simulink model "Simple_4Quad_payload_08_2017b"  (R2017b)
settings: Solver=ode45  StartTime=0.0  StopTime=200  RelTol=1e-3
InitFcn:
  | Simple_4Quad_payload_08_const
values from neighbouring files (symbols this model uses):
  All_rho = [d1 0 0 ... (first row only)    [Colab_4Quad_model_01_const.m]    (also in Colab_4Quad_model_02_const.m; Simple_4Quad_payload_04_const.m; Simple_4Quad_payload_05_const.m; Simple_4Quad_payload_06_const.m)
  alphaTF = 0.1    [Simple_4Quad_payload_08_const.m]    (also in Simple_4Quad_payload_09_const.m = 0.5; Simple_4Quad_payload_10_const.m = 1; Simple_4Quad_payload_11_const.m = 0.5; Simple_4Quad_payload_12_const.m = 10)
  B_ob = [zeros(3);eye(3)]    [Simple_4Quad_payload_04_const.m]    (also in Simple_4Quad_payload_05_const.m; Simple_4Quad_payload_06_const.m; Simple_4Quad_payload_07_const.m; Simple_4Quad_payload_08_const.m)
  BBT_inv = ((B'*B)^(-1))*B'    [Simple_2Quad_payload_03_const.m]    (also in Simple_4Quad_payload_04_const.m = ((BR'*BR)^(-1))*BR'; Simple_4Quad_payload_05_const.m = ((BR'*BR)^(-1))*BR'; Simple_4Quad_payload_06_const.m = ((BR'*BR)^(-1))*BR'; Simple_4Quad_payload_07_const.m = ((BR'*BR)^(-1))*BR')
  BR = 1e0*eye(n)    [Simple_4Quad_payload_04_const.m]    (also in Simple_4Quad_payload_05_const.m; Simple_4Quad_payload_06_const.m; Simple_4Quad_payload_07_const.m; Simple_4Quad_payload_08_const.m)
  C_ob = [eye(3) zeros(3)]    [Simple_4Quad_payload_04_const.m]    (also in Simple_4Quad_payload_05_const.m; Simple_4Quad_payload_06_const.m; Simple_4Quad_payload_07_const.m; Simple_4Quad_payload_08_const.m)
  d1 = 0.25    [Colab_4Quad_model_01_const.m]    (also in Colab_4Quad_model_02_const.m = 0.5; Simple_4Quad_payload_01_const.m = 1; Simple_4Quad_payload_02_const.m = 1; Simple_4Quad_payload_03_const.m = 1)
  d2 = 0.25    [Colab_4Quad_model_01_const.m]    (also in Colab_4Quad_model_02_const.m = 0.5; Simple_4Quad_payload_01_const.m = 1; Simple_4Quad_payload_02_const.m = 1; Simple_4Quad_payload_03_const.m = 1)
  Des_rel_dist = 2    [Simple_4Quad_payload_01_const.m]    (also in Simple_4Quad_payload_02_const.m = 4; Simple_4Quad_payload_03_const.m = 4; Simple_4Quad_payload_04_const.m; Simple_4Quad_payload_05_const.m)
  g = 9.81    [Colab_4Quad_model_01_const.m]    (also in Colab_4Quad_model_02_const.m; Simple_2Quad_payload_01_const.m; Simple_2Quad_payload_02_const.m; Simple_2Quad_payload_03_const.m)
  gamma_0 = 1e-0*diag([1e-3;1e-0])    [Simple_2Quad_payload_03_const.m]    (also in Simple_4Quad_payload_04_const.m = 1e-0*diag([1e-6*ones(3,1);1e-0*ones(3,1)]); Simple_4Quad_payload_05_const.m = 1e-1*diag([1e-6*ones(3,1);1e-0*ones(3,1)]); Simple_4Quad_payload_06_const.m = 1e-0*diag([1e-6*ones(3,1);1e-0*ones(3,1)]); Simple_4Quad_payload_07_const.m = 1e-0*diag([1e-6*ones(3,1);1e-0*ones(3,1)]))
  gamma_0L = 1e-0*diag([1e-6*ones(3,1);1e-0*ones(3,1)])    [Simple_4Quad_payload_08_const.m]    (also in Simple_4Quad_payload_09_const.m; Simple_4Quad_payload_10_const.m = 1e+0*diag([1e-3*ones(3,1);1e-3*ones(3,1)]); Simple_4Quad_payload_11_const.m = 1e+0*diag([1e-3*ones(3,1);1e-3*ones(3,1)]); Simple_4Quad_payload_12_const.m = 1e+2*diag(1e-4*ones(3,1)))
  gamma_0o = 1e-6*diag([1e-0*ones(3,1);1e-0*ones(3,1)])    [Simple_4Quad_payload_08_const.m]    (also in Simple_4Quad_payload_09_const.m = 1e-0*diag([1e-3*ones(3,1);1e-3*ones(3,1)]))
  gamma_0v = 1e-0*diag([1e-0*ones(3,1);1e-0*ones(3,1)])    [Simple_4Quad_payload_08_const.m]    (also in Simple_4Quad_payload_09_const.m = 1e-0*diag([1e-6*ones(3,1);1e-6*ones(3,1)]); Simple_4Quad_payload_10_const.m = 1e+0*diag(1e-0*ones(3,1)); Simple_4Quad_payload_11_const.m = 1e+0*diag(1e-0*ones(3,1)); Simple_4Quad_payload_12_const.m = 1e+3*diag(1e-0*ones(3,1)))
  gamma_1 = 1e+2*diag([1e-3;1e-0])    [Simple_2Quad_payload_03_const.m]    (also in Simple_4Quad_payload_04_const.m = 1e+2*diag([1e-6*ones(3,1);1e-0*ones(3,1)]); Simple_4Quad_payload_05_const.m = 1e+2*diag([1e-6*ones(3,1);1e-0*ones(3,1)]); Simple_4Quad_payload_06_const.m = 1e+3*diag([1e-6*ones(3,1);1e-0*ones(3,1)]); Simple_4Quad_payload_07_const.m = 1e+3*diag([1e-6*ones(3,1);1e-0*ones(3,1)]))
  gamma_1L = 1e+3*diag([1e-6*ones(3,1);1e-0*ones(3,1)])    [Simple_4Quad_payload_08_const.m]    (also in Simple_4Quad_payload_09_const.m = 1e+2*diag([1e-6*ones(3,1);1e-0*ones(3,1)]); Simple_4Quad_payload_10_const.m = 1e+1*diag([1e-3*ones(3,1);1e-3*ones(3,1)]); Simple_4Quad_payload_11_const.m = 1e+0*diag([1e-3*ones(3,1);1e-3*ones(3,1)]); Simple_4Quad_payload_12_const.m = 1e+2*diag(1e-4*ones(3,1)))
  gamma_1o = 1e-6*diag([1e-0*ones(3,1);1e-0*ones(3,1)])    [Simple_4Quad_payload_08_const.m]    (also in Simple_4Quad_payload_09_const.m = 1e+2*diag([1e-3*ones(3,1);1e-3*ones(3,1)]))
  gamma_1v = 1e+3*diag([1e-0*ones(3,1);1e-0*ones(3,1)])    [Simple_4Quad_payload_08_const.m]    (also in Simple_4Quad_payload_09_const.m = 1e+2*diag([1e-6*ones(3,1);1e-6*ones(3,1)]); Simple_4Quad_payload_10_const.m = 1e+0*diag(1e-0*ones(3,1)); Simple_4Quad_payload_11_const.m = 1e+0*diag(1e-0*ones(3,1)); Simple_4Quad_payload_12_const.m = 1e+3*diag(1e-0*ones(3,1)))
  Ix = 0.166667    [Colab_4Quad_model_01_const.m]    (also in Colab_4Quad_model_02_const.m = 0.02; Simple_4Quad_payload_01_const.m = 1; Simple_4Quad_payload_02_const.m = 1; Simple_4Quad_payload_03_const.m = 1)
  Iy = 0.166667    [Colab_4Quad_model_01_const.m]    (also in Colab_4Quad_model_02_const.m = 0.02; Simple_4Quad_payload_01_const.m = 1; Simple_4Quad_payload_02_const.m = 1; Simple_4Quad_payload_03_const.m = 1)
  Iz = 0.166667    [Colab_4Quad_model_01_const.m]    (also in Colab_4Quad_model_02_const.m = 0.02; Simple_4Quad_payload_01_const.m = 1; Simple_4Quad_payload_02_const.m = 1; Simple_4Quad_payload_03_const.m = 1)
  Jo = diag([Ix;Iy;Iz])    [Colab_4Quad_model_01_const.m]    (also in Colab_4Quad_model_02_const.m; Simple_4Quad_payload_04_const.m; Simple_4Quad_payload_05_const.m; Simple_4Quad_payload_06_const.m)
  Jq = diag([0.0291 0.0291 0.0552])    [Colab_4Quad_model_01_const.m]    (also in Colab_4Quad_model_02_const.m = diag([0.03 0.03 0.06]); Simple_4Quad_payload_03_const.m = 1.2416e-3 * diag([1 1 2]); Simple_4Quad_payload_04_const.m = 1 * diag([1 1 2]); Simple_4Quad_payload_05_const.m = 1 * diag([1 1 2]))
  k1 = 1    [Simple_2Quad_payload_03_const.m]    (also in Simple_4Quad_payload_04_const.m; Simple_4Quad_payload_05_const.m; Simple_4Quad_payload_06_const.m; Simple_4Quad_payload_07_const.m)
  k2 = 0.1    [Simple_2Quad_payload_03_const.m]    (also in Simple_4Quad_payload_04_const.m; Simple_4Quad_payload_05_const.m; Simple_4Quad_payload_06_const.m; Simple_4Quad_payload_07_const.m)
  l = 3.1819    [Colab_4Quad_model_01_const.m]    (also in Colab_4Quad_model_02_const.m = 3; Simple_2Quad_payload_04_const.m = 1; Simple_4Quad_payload_01_const.m = 1; Simple_4Quad_payload_02_const.m = 2)
  m = 1.5    [Colab_4Quad_model_01_const.m]    (also in Colab_4Quad_model_02_const.m; Simple_2Quad_payload_04_const.m = 1; Simple_4Quad_payload_01_const.m = 1; Simple_4Quad_payload_02_const.m = 1)
  M = 1.0    (= 1)    [Colab_4Quad_model_01_const.m]    (also in Colab_4Quad_model_02_const.m; Simple_2Quad_payload_01_const.m; Simple_2Quad_payload_02_const.m; Simple_2Quad_payload_03_const.m)
  n = 2    [Simple_2Quad_payload_03_const.m]    (also in Simple_4Quad_payload_03_const.m = 6; Simple_4Quad_payload_04_const.m = 6; Simple_4Quad_payload_05_const.m = 6; Simple_4Quad_payload_06_const.m = 6)
  noise_var_Omegao = 0e-6    (= 0)    [Simple_4Quad_payload_07_const.m]    (also in Simple_4Quad_payload_08_const.m; Simple_4Quad_payload_09_const.m; Simple_4Quad_payload_10_const.m; Simple_4Quad_payload_11_const.m)
  noise_var_RelAcc = 0e-6    (= 0)    [Simple_4Quad_payload_07_const.m]    (also in Simple_4Quad_payload_08_const.m; Simple_4Quad_payload_09_const.m; Simple_4Quad_payload_10_const.m; Simple_4Quad_payload_11_const.m)
  noise_var_RelPos = 0e-6    (= 0)    [Simple_4Quad_payload_07_const.m]    (also in Simple_4Quad_payload_08_const.m; Simple_4Quad_payload_09_const.m; Simple_4Quad_payload_10_const.m; Simple_4Quad_payload_11_const.m)
  Q_ob = var_u_ob * eye(6)    [Simple_4Quad_payload_04_const.m]    (also in Simple_4Quad_payload_05_const.m; Simple_4Quad_payload_06_const.m; Simple_4Quad_payload_07_const.m; Simple_4Quad_payload_08_const.m)
  QL = 1e-0*eye(n)    [Simple_4Quad_payload_08_const.m]    (also in Simple_4Quad_payload_09_const.m; Simple_4Quad_payload_10_const.m; Simple_4Quad_payload_11_const.m = 1e-2*eye(n); Simple_4Quad_payload_12_const.m = 1e-0*eye(np))
  Qo = 1e-0*eye(n)    [Simple_4Quad_payload_08_const.m]    (also in Simple_4Quad_payload_09_const.m)
  QR = 1e-0*eye(n)    [Simple_4Quad_payload_04_const.m]    (also in Simple_4Quad_payload_05_const.m = 1e-1*eye(n); Simple_4Quad_payload_06_const.m; Simple_4Quad_payload_07_const.m; Simple_4Quad_payload_08_const.m)
  Qv = 1e-0*eye(n)    [Simple_4Quad_payload_08_const.m]    (also in Simple_4Quad_payload_09_const.m; Simple_4Quad_payload_10_const.m = 1e-0*eye(np); Simple_4Quad_payload_11_const.m = 1e-2*eye(np); Simple_4Quad_payload_12_const.m = 1e-0*eye(np))
  R = 1e+0*eye(n)    [Simple_2Quad_payload_03_const.m]    (also in Simple_4Quad_payload_04_const.m = 1e+0*eye(m); Simple_4Quad_payload_05_const.m = 1e+0*eye(m); Simple_4Quad_payload_06_const.m; Simple_4Quad_payload_07_const.m)
  R_ob = var_y_ob * eye(3)    [Simple_4Quad_payload_04_const.m]    (also in Simple_4Quad_payload_05_const.m; Simple_4Quad_payload_06_const.m; Simple_4Quad_payload_07_const.m; Simple_4Quad_payload_08_const.m)
  rho_0 = 1e-0    (= 1)    [Simple_2Quad_payload_03_const.m]    (also in Simple_4Quad_payload_04_const.m; Simple_4Quad_payload_05_const.m = 0.1; Simple_4Quad_payload_06_const.m; Simple_4Quad_payload_07_const.m)
  rho_0L = 1e-0    (= 1)    [Simple_4Quad_payload_08_const.m]    (also in Simple_4Quad_payload_09_const.m; Simple_4Quad_payload_10_const.m; Simple_4Quad_payload_11_const.m; Simple_4Quad_payload_12_const.m)
  rho_0o = 1e-1    (= 0.1)    [Simple_4Quad_payload_08_const.m]    (also in Simple_4Quad_payload_09_const.m = 1)
  rho_0v = 1e-1    (= 0.1)    [Simple_4Quad_payload_08_const.m]    (also in Simple_4Quad_payload_09_const.m = 1; Simple_4Quad_payload_10_const.m = 1; Simple_4Quad_payload_11_const.m = 1; Simple_4Quad_payload_12_const.m = 1)
  rho_1 = 1e-0    (= 1)    [Simple_2Quad_payload_03_const.m]    (also in Simple_4Quad_payload_04_const.m; Simple_4Quad_payload_05_const.m; Simple_4Quad_payload_06_const.m; Simple_4Quad_payload_07_const.m)
  rho_1L = 1e-0    (= 1)    [Simple_4Quad_payload_08_const.m]    (also in Simple_4Quad_payload_09_const.m; Simple_4Quad_payload_10_const.m; Simple_4Quad_payload_11_const.m; Simple_4Quad_payload_12_const.m)
  rho_1o = 1e-0    (= 1)    [Simple_4Quad_payload_08_const.m]    (also in Simple_4Quad_payload_09_const.m)
  rho_1v = 1e-0    (= 1)    [Simple_4Quad_payload_08_const.m]    (also in Simple_4Quad_payload_09_const.m; Simple_4Quad_payload_10_const.m; Simple_4Quad_payload_11_const.m; Simple_4Quad_payload_12_const.m)
(part 2 of 4)

== system Simple_4Quad_payload_08_2017b/Dynamic model of the entire system/Control inputs from Q1 ==
  Omega_Q1 : Inport
  U1_local_paral_INP : Inport  Port=2
  U1_local_perpn_INP : Inport  Port=3
  q1 : Inport  Port=4
  UT1 : Inport  Port=5
  PHIo : Inport  Port=6
  Controller Interpreter #2 : MATLAB Function  TreatAsAtomicUnit=on
  Demux : Demux  Outputs=3
  Demux1 : Demux  Outputs=3
  Rotation_Q1 : Subsystem
  Scope : Scope  NumInputPorts=3
  Scope1 : Scope  NumInputPorts=3
  U1_local_paral_OUT : Outport
  U1_local_perpn_OUT : Outport  Port=2
  X_ROT_Q1 : Outport  Port=3
  tag scope: PHI_1=global, U1_local_paral_ACT=global, U1_local_perpn_ACT=global
  wires:
  UT1/1 -> Controller Interpreter #2/1(UTi)
  q1/1 -> Controller Interpreter #2/2(qi)
  Omega_Q1/1 -> Rotation_Q1/1(Omega Q1)
  Rotation_Q1/1(X_Rot_Q1) -> X_ROT_Q1/1
  PHIo/1 -> Controller Interpreter #2/4(PHIo)
  Controller Interpreter #2/2(Ui_local_perpn) -> U1_local_perpn_OUT/1, [U1_local_perpn_ACT]
  Controller Interpreter #2/1(Ui_local_paral) -> U1_local_paral_OUT/1, [U1_local_paral_ACT]
  [PHI_d1] -> Demux1/1
  Demux/1 -> Scope/1
  Demux/2 -> Scope/2
  Demux/3 -> Scope/3
  Demux1/3 -> Scope1/3
  Demux1/2 -> Scope1/2
  Demux1/1 -> Scope1/1
  Rotation_Q1/2(PHI_Q1) -> [PHI_1], Controller Interpreter #2/3(PHIi), Demux/1

== system Simple_4Quad_payload_08_2017b/Dynamic model of the entire system/Control inputs from Q2 ==
  Omega_Q2 : Inport
  U2_local_paral_INP : Inport  Port=2
  U2_local_perpn_INP : Inport  Port=3
  q2 : Inport  Port=4
  UT2 : Inport  Port=5
  PHIo : Inport  Port=6
  Controller Interpreter #2 : MATLAB Function  TreatAsAtomicUnit=on
  Rotation_Q2 : Subsystem
  U2_local_paral_OUT : Outport
  U2_local_perpn_OUT : Outport  Port=2
  X_ROT_Q2 : Outport  Port=3
  tag scope: PHI_2=global, U2_local_paral_ACT=global, U2_local_perpn_ACT=global
  wires:
  PHIo/1 -> Controller Interpreter #2/4(PHIo)
  Rotation_Q2/1(X_Rot_Q2) -> X_ROT_Q2/1
  Omega_Q2/1 -> Rotation_Q2/1(Omega Q2)
  q2/1 -> Controller Interpreter #2/2(qi)
  UT2/1 -> Controller Interpreter #2/1(UTi)
  Controller Interpreter #2/2(Ui_local_perpn) -> U2_local_perpn_OUT/1, [U2_local_perpn_ACT]
  Controller Interpreter #2/1(Ui_local_paral) -> U2_local_paral_OUT/1, [U2_local_paral_ACT]
  Rotation_Q2/2(PHI_Q2) -> [PHI_2], Controller Interpreter #2/3(PHIi)

== system Simple_4Quad_payload_08_2017b/Dynamic model of the entire system/Control inputs from Q3 ==
  Omega_Q3 : Inport
  U3_local_paral_INP : Inport  Port=2
  U3_local_perpn_INP : Inport  Port=3
  q3 : Inport  Port=4
  UT3 : Inport  Port=5
  PHIo : Inport  Port=6
  Controller Interpreter #2 : MATLAB Function  TreatAsAtomicUnit=on
  Rotation_Q3 : Subsystem
  U3_local_paral_OUT : Outport
  U3_local_perpn_OUT : Outport  Port=2
  X_ROT_Q3 : Outport  Port=3
  tag scope: PHI_3=global, U3_local_paral_ACT=global, U3_local_perpn_ACT=global
  wires:
  UT3/1 -> Controller Interpreter #2/1(UTi)
  q3/1 -> Controller Interpreter #2/2(qi)
  Omega_Q3/1 -> Rotation_Q3/1(Omega Q3)
  Rotation_Q3/1(X_Rot_Q3) -> X_ROT_Q3/1
  PHIo/1 -> Controller Interpreter #2/4(PHIo)
  Controller Interpreter #2/2(Ui_local_perpn) -> U3_local_perpn_OUT/1, [U3_local_perpn_ACT]
  Controller Interpreter #2/1(Ui_local_paral) -> U3_local_paral_OUT/1, [U3_local_paral_ACT]
  Rotation_Q3/2(PHI_Q3) -> [PHI_3], Controller Interpreter #2/3(PHIi)

== system Simple_4Quad_payload_08_2017b/Dynamic model of the entire system/Control inputs from Q4 ==
  Omega_Q4 : Inport
  U4_local_paral_INP : Inport  Port=2
  U4_local_perpn_INP : Inport  Port=3
  q4 : Inport  Port=4
  UT4 : Inport  Port=5
  PHIo : Inport  Port=6
  Controller Interpreter #2 : MATLAB Function  TreatAsAtomicUnit=on
  Rotation_Q4 : Subsystem
  U4_local_paral_OUT : Outport
  U4_local_perpn_OUT : Outport  Port=2
  X_ROT_Q4 : Outport  Port=3
  tag scope: PHI_4=global, U4_local_paral_ACT=global, U4_local_perpn_ACT=global
  wires:
  PHIo/1 -> Controller Interpreter #2/4(PHIo)
  Rotation_Q4/1(X_Rot_Q4) -> X_ROT_Q4/1
  Omega_Q4/1 -> Rotation_Q4/1(Omega Q4)
  q4/1 -> Controller Interpreter #2/2(qi)
  UT4/1 -> Controller Interpreter #2/1(UTi)
  Controller Interpreter #2/1(Ui_local_paral) -> U4_local_paral_OUT/1, [U4_local_paral_ACT]
  Rotation_Q4/2(PHI_Q4) -> Controller Interpreter #2/3(PHIi), [PHI_4]
  Controller Interpreter #2/2(Ui_local_perpn) -> U4_local_perpn_OUT/1, [U4_local_perpn_ACT]

== system Simple_4Quad_payload_08_2017b/Rotational Controller Log/For matrix Plot ==
  P : Inport
  MATLAB Function : MATLAB Function  TreatAsAtomicUnit=on
  To Workspace : ToWorkspace  VariableName=P1_R  SaveFormat=Structure With Time  SampleTime=-1
  wires:
  MATLAB Function/1(y) -> To Workspace/1
  P/1 -> MATLAB Function/1(u)

== system Simple_4Quad_payload_08_2017b/Rotational Controller Log/For matrix Plot1 ==
  P : Inport
  MATLAB Function : MATLAB Function  TreatAsAtomicUnit=on
  To Workspace : ToWorkspace  VariableName=P2_R  SaveFormat=Structure With Time  SampleTime=-1
  wires:
  P/1 -> MATLAB Function/1(u)
  MATLAB Function/1(y) -> To Workspace/1

== system Simple_4Quad_payload_08_2017b/Rotational Controller Log/For matrix Plot2 ==
  P : Inport
  MATLAB Function : MATLAB Function  TreatAsAtomicUnit=on
  To Workspace : ToWorkspace  VariableName=P3_R  SaveFormat=Structure With Time  SampleTime=-1
  wires:
  P/1 -> MATLAB Function/1(u)
  MATLAB Function/1(y) -> To Workspace/1

== system Simple_4Quad_payload_08_2017b/Rotational Controller Log/For matrix Plot3 ==
  P : Inport
  MATLAB Function : MATLAB Function  TreatAsAtomicUnit=on
  To Workspace : ToWorkspace  VariableName=P4_R  SaveFormat=Structure With Time  SampleTime=-1
  wires:
  MATLAB Function/1(y) -> To Workspace/1
  P/1 -> MATLAB Function/1(u)

== system Simple_4Quad_payload_08_2017b/Rotational Controller Log/For matrix Plot4 ==
  A_hat : Inport
  MATLAB Function : MATLAB Function  TreatAsAtomicUnit=on
  To Workspace : ToWorkspace  VariableName=A_hat1_R  SaveFormat=Structure With Time  SampleTime=-1
  wires:
  A_hat/1 -> MATLAB Function/1(u)
  MATLAB Function/1(y) -> To Workspace/1

== system Simple_4Quad_payload_08_2017b/Rotational Controller Log/For matrix Plot5 ==
  A_hat : Inport
  MATLAB Function : MATLAB Function  TreatAsAtomicUnit=on
  To Workspace : ToWorkspace  VariableName=A_hat2_R  SaveFormat=Structure With Time  SampleTime=-1
  wires:
  MATLAB Function/1(y) -> To Workspace/1
  A_hat/1 -> MATLAB Function/1(u)

== system Simple_4Quad_payload_08_2017b/Rotational Controller Log/For matrix Plot6 ==
  A_hat : Inport
  MATLAB Function : MATLAB Function  TreatAsAtomicUnit=on
  To Workspace : ToWorkspace  VariableName=A_hat3_R  SaveFormat=Structure With Time  SampleTime=-1
  wires:
  A_hat/1 -> MATLAB Function/1(u)
  MATLAB Function/1(y) -> To Workspace/1

== system Simple_4Quad_payload_08_2017b/Rotational Controller Log/For matrix Plot7 ==
  A_hat : Inport
  MATLAB Function : MATLAB Function  TreatAsAtomicUnit=on
  To Workspace : ToWorkspace  VariableName=A_hat4_R  SaveFormat=Structure With Time  SampleTime=-1
  wires:
  MATLAB Function/1(y) -> To Workspace/1
  A_hat/1 -> MATLAB Function/1(u)

== system Simple_4Quad_payload_08_2017b/Controllers and Observers/Controlelr and Observer - Agent3/Link #3 ==
  x_rd : Inport
  X : Inport  Port=2
  CARE : MATLAB Function  TreatAsAtomicUnit=on
  Differentiator : Subsystem
  Integrator : Integrator  InitialCondition=zeros(n)
  Integrator1 : Integrator  InitialCondition=eye(n)
  Integrator2 : Integrator  InitialCondition=zeros(n,1)
  Integrator3 : Integrator  ExternalReset=level  InitialCondition=zeros(n,1)
  Memory : Memory  InitialCondition=zeros(n,1)
  Memory1 : Memory  InitialCondition=zeros(3,1)
  Sum : Sum  Inputs=|++
  g-Estimator : MATLAB Function  TreatAsAtomicUnit=on
  g-Estimator1 : MATLAB Function  TreatAsAtomicUnit=on
  main : MATLAB Function  TreatAsAtomicUnit=on
  output definition : MATLAB Function  TreatAsAtomicUnit=on
  variable change : MATLAB Function  TreatAsAtomicUnit=on
  N3 : Outport
  wires:
  x_rd/1 -> variable change/2(Xd)
  X/1 -> variable change/1(X)
  CARE/1(DP) -> Integrator1/1
  Sum/1 -> main/1(sigma), g-Estimator/1(sigma), g-Estimator1/1(sigma)
  g-Estimator1/1(Da_hat) -> Integrator/1
  variable change/1(x_mod) -> main/7(x), g-Estimator1/2(x)
  Integrator1/1 -> g-Estimator1/3(P), CARE/1(P), g-Estimator/3(P), main/4(P)
  Integrator/1 -> g-Estimator1/4(a_hat), CARE/2(a_hat), main/5(a_hat)
  g-Estimator/1(Dg_hat) -> Integrator2/1
  Differentiator/1(Dx_d) -> main/3(Dy_d)
  Integrator3/1 -> main/2(zeta), Sum/1
  variable change/2(xd_mod) -> Differentiator/1(x_d)
  variable change/3(e_mod) -> Sum/2, Integrator3/2, Integrator3/1
  Integrator2/1 -> main/6(g_hat), g-Estimator/2(g_hat)
  output definition/1(ur) -> Memory1/1
  Memory1/1 -> N3/1
  main/1(u) -> output definition/1(u), Memory/1
  Memory/1 -> variable change/3(u)

== system Simple_4Quad_payload_08_2017b/Controllers and Observers/Controlelr and Observer - Agent3/Observer3 ==
  wo : Inport
  Dwo : Inport  Port=2
  Rel_Pos_local3 : Inport  Port=3
  Rel_Acc_local3 : Inport  Port=4
  Agent_Num : Inport  Port=5
  Integrator : Integrator  InitialCondition=eye(6)
  Integrator1 : Integrator  InitialCondition=[0;0;1;0;0;0]
  Kalman_Filter3 : MATLAB Function  TreatAsAtomicUnit=on
  Observer_Finalization3 : MATLAB Function  TreatAsAtomicUnit=on
  q3_hat : Outport
  Dq3_hat : Outport  Port=2
  tag scope: Dq3_hat=global, q3_hat=global
  wires:
  Kalman_Filter3/1(DP_ob) -> Integrator/1
  Kalman_Filter3/2(Dxhat_ob) -> Integrator1/1
  Integrator/1 -> Kalman_Filter3/1(P_ob)
  Integrator1/1 -> Observer_Finalization3/1(xhati), Kalman_Filter3/2(xhat_ob)
  wo/1 -> Kalman_Filter3/3(wo)
  Dwo/1 -> Kalman_Filter3/4(Dwo)
  Rel_Pos_local3/1 -> Kalman_Filter3/5(Rel_Posi_local)
  Rel_Acc_local3/1 -> Kalman_Filter3/6(Rel_Acci_local)
  Agent_Num/1 -> Kalman_Filter3/7(Agent_Num)
  Observer_Finalization3/1(qhati) -> [q3_hat], q3_hat/1
  Observer_Finalization3/2(Dqhati) -> [Dq3_hat], Dq3_hat/1

== system Simple_4Quad_payload_08_2017b/Controllers and Observers/Controlelr and Observer - Agent3/Rotational #3 ==
  x_rd : Inport
  X : Inport  Port=2
  CARE : MATLAB Function  TreatAsAtomicUnit=on
  Differentiator : Subsystem
  Integrator : Integrator  InitialCondition=zeros(n)
  Integrator1 : Integrator  InitialCondition=eye(n)
  Integrator2 : Integrator  InitialCondition=zeros(n,1)
  Integrator3 : Integrator  InitialCondition=zeros(n,1)
  Memory : Memory  InitialCondition=zeros(n,1)
  Memory1 : Memory  InitialCondition=zeros(3,1)
  Scope10 : Scope
  Sum : Sum  Inputs=|++
  g-Estimator : MATLAB Function  TreatAsAtomicUnit=on
  g-Estimator1 : MATLAB Function  TreatAsAtomicUnit=on
  main : MATLAB Function  TreatAsAtomicUnit=on
  output definition : MATLAB Function  TreatAsAtomicUnit=on
  variable change : MATLAB Function  TreatAsAtomicUnit=on
  ur : Outport
  tag scope: A_hat3_R=global, P3_R=global, e3_R=global, g_hat3_R=global
  wires:
  Integrator2/1 -> g-Estimator/2(g_hat), [g_hat3_R], main/6(g_hat)
  Memory/1 -> variable change/3(u)
  variable change/3(e_mod) -> Integrator3/1, Sum/2, [e3_R]
  variable change/2(xd_mod) -> Differentiator/1(x_d)
  Integrator3/1 -> Sum/1, main/2(zeta)
  main/1(u) -> output definition/1(u), Memory/1
  Differentiator/1(Dx_d) -> main/3(Dy_d)
  g-Estimator/1(Dg_hat) -> Integrator2/1
  Integrator/1 -> main/5(a_hat), CARE/2(a_hat), g-Estimator1/4(a_hat), [A_hat3_R]
  Integrator1/1 -> main/4(P), g-Estimator/3(P), [P3_R], CARE/1(P), g-Estimator1/3(P)
  variable change/1(x_mod) -> g-Estimator1/2(x), main/7(x)
  g-Estimator1/1(Da_hat) -> Integrator/1
  Sum/1 -> g-Estimator1/1(sigma), g-Estimator/1(sigma), Scope10/1, main/1(sigma)
  CARE/1(DP) -> Integrator1/1
  X/1 -> variable change/1(X)
  x_rd/1 -> variable change/2(Xd)
  output definition/1(ur) -> Memory1/1
  Memory1/1 -> ur/1

== system Simple_4Quad_payload_08_2017b/Controllers and Observers/Controller - Payload/Payload ==
  x_rd : Inport
  X : Inport  Port=2
  CARE : MATLAB Function  TreatAsAtomicUnit=on
  Differentiator : Subsystem
  Integrator : Integrator  InitialCondition=zeros(n)
  Integrator1 : Integrator  InitialCondition=eye(n)
  Integrator2 : Integrator  InitialCondition=zeros(n,1)
  Integrator3 : Integrator  ExternalReset=level  InitialCondition=zeros(n,1)
  Sum : Sum  Inputs=|++
  g-Estimator : MATLAB Function  TreatAsAtomicUnit=on
  g-Estimator1 : MATLAB Function  TreatAsAtomicUnit=on
  main : MATLAB Function  TreatAsAtomicUnit=on
  variable change : MATLAB Function  TreatAsAtomicUnit=on
  z : Outport
  wires:
  x_rd/1 -> variable change/2(Xd)
  X/1 -> variable change/1(X)
  CARE/1(DP) -> Integrator1/1
  Sum/1 -> main/1(sigma), g-Estimator/1(sigma), g-Estimator1/1(sigma)
  g-Estimator1/1(Da_hat) -> Integrator/1
  variable change/1(x_mod) -> main/7(x), g-Estimator1/2(x)
  Integrator1/1 -> g-Estimator1/3(P), CARE/1(P), g-Estimator/3(P), main/4(P)
  Integrator/1 -> g-Estimator1/4(a_hat), CARE/2(a_hat), main/5(a_hat)
  g-Estimator/1(Dg_hat) -> Integrator2/1
  Differentiator/1(Dx_d) -> main/3(Dy_d)
  Integrator3/1 -> main/2(zeta), Sum/1
  variable change/2(xd_mod) -> Differentiator/1(x_d)
  variable change/3(e_mod) -> Sum/2, Integrator3/2, Integrator3/1
  Integrator2/1 -> main/6(g_hat), g-Estimator/2(g_hat)
  main/1(u) -> z/1

== system Simple_4Quad_payload_08_2017b/Controllers and Observers/Controller - Payload/Payload1 ==
  x_rd : Inport
  X : Inport  Port=2
  CARE : MATLAB Function  TreatAsAtomicUnit=on
  Differentiator : Subsystem
  Integrator : Integrator  InitialCondition=zeros(n)
  Integrator1 : Integrator  InitialCondition=eye(n)
  Integrator2 : Integrator  InitialCondition=zeros(n,1)
  Integrator3 : Integrator  ExternalReset=level  InitialCondition=zeros(n,1)
  Sum : Sum  Inputs=|++
  g-Estimator : MATLAB Function  TreatAsAtomicUnit=on
  g-Estimator1 : MATLAB Function  TreatAsAtomicUnit=on
  main : MATLAB Function  TreatAsAtomicUnit=on
  variable change : MATLAB Function  TreatAsAtomicUnit=on
  z : Outport
  wires:
  x_rd/1 -> variable change/2(Xd)
  X/1 -> variable change/1(X)
  CARE/1(DP) -> Integrator1/1
  Sum/1 -> main/1(sigma), g-Estimator/1(sigma), g-Estimator1/1(sigma)
  g-Estimator1/1(Da_hat) -> Integrator/1
  variable change/1(x_mod) -> main/7(x), g-Estimator1/2(x)
  Integrator1/1 -> g-Estimator1/3(P), CARE/1(P), g-Estimator/3(P), main/4(P)
  Integrator/1 -> g-Estimator1/4(a_hat), CARE/2(a_hat), main/5(a_hat)
  g-Estimator/1(Dg_hat) -> Integrator2/1
  Differentiator/1(Dx_d) -> main/3(Dy_d)
  Integrator3/1 -> main/2(zeta), Sum/1
  variable change/2(xd_mod) -> Differentiator/1(x_d)
  variable change/3(e_mod) -> Sum/2, Integrator3/2, Integrator3/1
  Integrator2/1 -> main/6(g_hat), g-Estimator/2(g_hat)
  main/1(u) -> z/1

== system Simple_4Quad_payload_08_2017b/Controllers and Observers/Controller - Payload/Rotation_Q1 ==
  Omega_O : Inport
  PHI_O : Inport  Port=2
  D Phi : MATLAB Function  TreatAsAtomicUnit=on
  D_PHI_O : Outport
  wires:
  D Phi/1(D_PHI_O) -> D_PHI_O/1
  Omega_O/1 -> D Phi/1(Omega_O)
  PHI_O/1 -> D Phi/2(PHI_O)

== system Simple_4Quad_payload_08_2017b/Controllers and Observers/Controller - Payload/Subsystem ==
  In1 : Inport
  Demux : Demux  Outputs=3
  Mux : Mux  Inputs=3
  Transfer Fcn : TransferFcn  Numerator=[alphaTF]  Denominator=[1 alphaTF]
  Transfer Fcn1 : TransferFcn  Numerator=[alphaTF]  Denominator=[1 alphaTF]
  Transfer Fcn2 : TransferFcn  Numerator=[alphaTF]  Denominator=[1 alphaTF]
  Out1 : Outport
  wires:
  In1/1 -> Demux/1
  Demux/2 -> Transfer Fcn1/1
  Demux/1 -> Transfer Fcn/1
  Demux/3 -> Transfer Fcn2/1
  Transfer Fcn1/1 -> Mux/2
  Transfer Fcn/1 -> Mux/1
  Transfer Fcn2/1 -> Mux/3
  Mux/1 -> Out1/1

== system Simple_4Quad_payload_08_2017b/Controllers and Observers/Controller and Observer - Agent2/Link #2 ==
  x_rd : Inport
  X : Inport  Port=2
  CARE : MATLAB Function  TreatAsAtomicUnit=on
  Differentiator : Subsystem
  Integrator : Integrator  InitialCondition=zeros(n)
  Integrator1 : Integrator  InitialCondition=eye(n)
  Integrator2 : Integrator  InitialCondition=zeros(n,1)
  Integrator3 : Integrator  ExternalReset=level  InitialCondition=zeros(n,1)
  Memory : Memory  InitialCondition=zeros(n,1)
  Memory1 : Memory  InitialCondition=zeros(3,1)
  Sum : Sum  Inputs=|++
  g-Estimator : MATLAB Function  TreatAsAtomicUnit=on
  g-Estimator1 : MATLAB Function  TreatAsAtomicUnit=on
  main : MATLAB Function  TreatAsAtomicUnit=on
  output definition : MATLAB Function  TreatAsAtomicUnit=on
  variable change : MATLAB Function  TreatAsAtomicUnit=on
  N2 : Outport
  wires:
  x_rd/1 -> variable change/2(Xd)
  X/1 -> variable change/1(X)
  CARE/1(DP) -> Integrator1/1
  Sum/1 -> main/1(sigma), g-Estimator/1(sigma), g-Estimator1/1(sigma)
  g-Estimator1/1(Da_hat) -> Integrator/1
  variable change/1(x_mod) -> main/7(x), g-Estimator1/2(x)
  Integrator1/1 -> g-Estimator1/3(P), CARE/1(P), g-Estimator/3(P), main/4(P)
  Integrator/1 -> g-Estimator1/4(a_hat), CARE/2(a_hat), main/5(a_hat)
  g-Estimator/1(Dg_hat) -> Integrator2/1
  Differentiator/1(Dx_d) -> main/3(Dy_d)
  Integrator3/1 -> main/2(zeta), Sum/1
  variable change/2(xd_mod) -> Differentiator/1(x_d)
  variable change/3(e_mod) -> Sum/2, Integrator3/2, Integrator3/1
  Integrator2/1 -> main/6(g_hat), g-Estimator/2(g_hat)
  output definition/1(ur) -> Memory1/1
  Memory1/1 -> N2/1
  main/1(u) -> output definition/1(u), Memory/1
  Memory/1 -> variable change/3(u)

== system Simple_4Quad_payload_08_2017b/Controllers and Observers/Controller and Observer - Agent2/Observer2 ==
  wo : Inport
  Dwo : Inport  Port=2
  Rel_Pos_local2 : Inport  Port=3
  Rel_Acc_local2 : Inport  Port=4
  Agent_Num : Inport  Port=5
  Integrator : Integrator  InitialCondition=eye(6)
  Integrator1 : Integrator  InitialCondition=[0;0;1;0;0;0]
  Kalman_Filter2 : MATLAB Function  TreatAsAtomicUnit=on
  Observer_Finalization2 : MATLAB Function  TreatAsAtomicUnit=on
  q2_hat : Outport
  Dq2_hat : Outport  Port=2
  tag scope: Dq2_hat=global, q2_hat=global
  wires:
  Kalman_Filter2/1(DP_ob) -> Integrator/1
  Kalman_Filter2/2(Dxhat_ob) -> Integrator1/1
  Integrator/1 -> Kalman_Filter2/1(P_ob)
  Integrator1/1 -> Kalman_Filter2/2(xhat_ob), Observer_Finalization2/1(xhati)
  wo/1 -> Kalman_Filter2/3(wo)
  Dwo/1 -> Kalman_Filter2/4(Dwo)
  Rel_Pos_local2/1 -> Kalman_Filter2/5(Rel_Posi_local)
  Rel_Acc_local2/1 -> Kalman_Filter2/6(Rel_Acci_local)
  Agent_Num/1 -> Kalman_Filter2/7(Agent_Num)
  Observer_Finalization2/1(qhati) -> [q2_hat], q2_hat/1
  Observer_Finalization2/2(Dqhati) -> [Dq2_hat], Dq2_hat/1

== system Simple_4Quad_payload_08_2017b/Controllers and Observers/Controller and Observer - Agent2/Rotational #2 ==
  x_rd : Inport
  X : Inport  Port=2
  CARE : MATLAB Function  TreatAsAtomicUnit=on
  Differentiator : Subsystem
  Integrator : Integrator  InitialCondition=zeros(n)
  Integrator1 : Integrator  InitialCondition=eye(n)
  Integrator2 : Integrator  InitialCondition=zeros(n,1)
  Integrator3 : Integrator  InitialCondition=zeros(n,1)
  Memory : Memory  InitialCondition=zeros(n,1)
  Memory1 : Memory  InitialCondition=zeros(3,1)
  Scope10 : Scope
  Sum : Sum  Inputs=|++
  g-Estimator : MATLAB Function  TreatAsAtomicUnit=on
  g-Estimator1 : MATLAB Function  TreatAsAtomicUnit=on
  main : MATLAB Function  TreatAsAtomicUnit=on
  output definition : MATLAB Function  TreatAsAtomicUnit=on
  variable change : MATLAB Function  TreatAsAtomicUnit=on
  ur : Outport
  tag scope: A_hat2_R=global, P2_R=global, e2_R=global, g_hat2_R=global
  wires:
  x_rd/1 -> variable change/2(Xd)
  X/1 -> variable change/1(X)
  CARE/1(DP) -> Integrator1/1
  Sum/1 -> main/1(sigma), Scope10/1, g-Estimator/1(sigma), g-Estimator1/1(sigma)
  g-Estimator1/1(Da_hat) -> Integrator/1
  variable change/1(x_mod) -> main/7(x), g-Estimator1/2(x)
  Integrator1/1 -> g-Estimator1/3(P), CARE/1(P), [P2_R], g-Estimator/3(P), main/4(P)
  Integrator/1 -> [A_hat2_R], g-Estimator1/4(a_hat), CARE/2(a_hat), main/5(a_hat)
  g-Estimator/1(Dg_hat) -> Integrator2/1
  Differentiator/1(Dx_d) -> main/3(Dy_d)
  main/1(u) -> Memory/1, output definition/1(u)
  Integrator3/1 -> main/2(zeta), Sum/1
  variable change/2(xd_mod) -> Differentiator/1(x_d)
  variable change/3(e_mod) -> [e2_R], Sum/2, Integrator3/1
  Memory/1 -> variable change/3(u)
  Integrator2/1 -> main/6(g_hat), [g_hat2_R], g-Estimator/2(g_hat)
  output definition/1(ur) -> Memory1/1
  Memory1/1 -> ur/1

== system Simple_4Quad_payload_08_2017b/Controllers and Observers/Controller and Observer - Agent4/Link #4 ==
  x_rd : Inport
  X : Inport  Port=2
  CARE : MATLAB Function  TreatAsAtomicUnit=on
  Differentiator : Subsystem
  Integrator : Integrator  InitialCondition=zeros(n)
  Integrator1 : Integrator  InitialCondition=eye(n)
  Integrator2 : Integrator  InitialCondition=zeros(n,1)
  Integrator3 : Integrator  ExternalReset=level  InitialCondition=zeros(n,1)
  Memory : Memory  InitialCondition=zeros(n,1)
  Memory1 : Memory  InitialCondition=zeros(3,1)
  Sum : Sum  Inputs=|++
  g-Estimator : MATLAB Function  TreatAsAtomicUnit=on
  g-Estimator1 : MATLAB Function  TreatAsAtomicUnit=on
  main : MATLAB Function  TreatAsAtomicUnit=on
  output definition : MATLAB Function  TreatAsAtomicUnit=on
  variable change : MATLAB Function  TreatAsAtomicUnit=on
  N4 : Outport
  wires:
  x_rd/1 -> variable change/2(Xd)
  X/1 -> variable change/1(X)
  CARE/1(DP) -> Integrator1/1
  Sum/1 -> main/1(sigma), g-Estimator/1(sigma), g-Estimator1/1(sigma)
  g-Estimator1/1(Da_hat) -> Integrator/1
  variable change/1(x_mod) -> main/7(x), g-Estimator1/2(x)
  Integrator1/1 -> g-Estimator1/3(P), CARE/1(P), g-Estimator/3(P), main/4(P)
  Integrator/1 -> g-Estimator1/4(a_hat), CARE/2(a_hat), main/5(a_hat)
  g-Estimator/1(Dg_hat) -> Integrator2/1
  Differentiator/1(Dx_d) -> main/3(Dy_d)
  Integrator3/1 -> main/2(zeta), Sum/1
  variable change/2(xd_mod) -> Differentiator/1(x_d)
  variable change/3(e_mod) -> Sum/2, Integrator3/2, Integrator3/1
  Integrator2/1 -> main/6(g_hat), g-Estimator/2(g_hat)
  output definition/1(ur) -> Memory1/1
  Memory1/1 -> N4/1
  main/1(u) -> output definition/1(u), Memory/1
  Memory/1 -> variable change/3(u)

== system Simple_4Quad_payload_08_2017b/Controllers and Observers/Controller and Observer - Agent4/Observer4 ==
  wo : Inport
  Dwo : Inport  Port=2
  Rel_Pos_local4 : Inport  Port=3
  Rel_Acc_local4 : Inport  Port=4
  Agent_Num : Inport  Port=5
  Integrator : Integrator  InitialCondition=eye(6)
  Integrator1 : Integrator  InitialCondition=[0;0;1;0;0;0]
  Kalman_Filter4 : MATLAB Function  TreatAsAtomicUnit=on
  Observer_Finalization4 : MATLAB Function  TreatAsAtomicUnit=on
  q4_hat : Outport
  Dq4_hat : Outport  Port=2
  tag scope: Dq4_hat=global, q4_hat=global
  wires:
  Kalman_Filter4/1(DP_ob) -> Integrator/1
  Kalman_Filter4/2(Dxhat_ob) -> Integrator1/1
  Integrator/1 -> Kalman_Filter4/1(P_ob)
  Integrator1/1 -> Observer_Finalization4/1(xhati), Kalman_Filter4/2(xhat_ob)
  wo/1 -> Kalman_Filter4/3(wo)
  Dwo/1 -> Kalman_Filter4/4(Dwo)
  Rel_Pos_local4/1 -> Kalman_Filter4/5(Rel_Posi_local)
  Rel_Acc_local4/1 -> Kalman_Filter4/6(Rel_Acci_local)
  Agent_Num/1 -> Kalman_Filter4/7(Agent_Num)
  Observer_Finalization4/1(qhati) -> [q4_hat], q4_hat/1
  Observer_Finalization4/2(Dqhati) -> [Dq4_hat], Dq4_hat/1

== system Simple_4Quad_payload_08_2017b/Controllers and Observers/Controller and Observer - Agent4/Rotational #4 ==
  x_rd : Inport
  X : Inport  Port=2
  CARE : MATLAB Function  TreatAsAtomicUnit=on
  Differentiator : Subsystem
  Integrator : Integrator  InitialCondition=zeros(n)
  Integrator1 : Integrator  InitialCondition=eye(n)
  Integrator2 : Integrator  InitialCondition=zeros(n,1)
  Integrator3 : Integrator  InitialCondition=zeros(n,1)
  Memory : Memory  InitialCondition=zeros(n,1)
  Memory1 : Memory  InitialCondition=zeros(3,1)
  Scope10 : Scope
  Sum : Sum  Inputs=|++
  g-Estimator : MATLAB Function  TreatAsAtomicUnit=on
  g-Estimator1 : MATLAB Function  TreatAsAtomicUnit=on
  main : MATLAB Function  TreatAsAtomicUnit=on
  output definition : MATLAB Function  TreatAsAtomicUnit=on
  variable change : MATLAB Function  TreatAsAtomicUnit=on
  ur : Outport
  tag scope: A_hat4_R=global, P4_R=global, e4_R=global, g_hat4_R=global
  wires:
  x_rd/1 -> variable change/2(Xd)
  X/1 -> variable change/1(X)
  CARE/1(DP) -> Integrator1/1
  Sum/1 -> main/1(sigma), Scope10/1, g-Estimator/1(sigma), g-Estimator1/1(sigma)
  g-Estimator1/1(Da_hat) -> Integrator/1
  variable change/1(x_mod) -> main/7(x), g-Estimator1/2(x)
  Integrator1/1 -> g-Estimator1/3(P), CARE/1(P), [P4_R], g-Estimator/3(P), main/4(P)
  Integrator/1 -> [A_hat4_R], g-Estimator1/4(a_hat), CARE/2(a_hat), main/5(a_hat)
  g-Estimator/1(Dg_hat) -> Integrator2/1
  Differentiator/1(Dx_d) -> main/3(Dy_d)
  main/1(u) -> Memory/1, output definition/1(u)
  Integrator3/1 -> main/2(zeta), Sum/1
  variable change/2(xd_mod) -> Differentiator/1(x_d)
  variable change/3(e_mod) -> [e4_R], Sum/2, Integrator3/1
  Memory/1 -> variable change/3(u)
  Integrator2/1 -> main/6(g_hat), [g_hat4_R], g-Estimator/2(g_hat)
  output definition/1(ur) -> Memory1/1
  Memory1/1 -> ur/1

== system Simple_4Quad_payload_08_2017b/Controllers and Observers/Cotnroller and Observer - Agent1 /Link #1 ==
  x_rd : Inport
  X : Inport  Port=2
  CARE : MATLAB Function  TreatAsAtomicUnit=on
  Differentiator : Subsystem
  Integrator : Integrator  InitialCondition=zeros(n)
  Integrator1 : Integrator  InitialCondition=eye(n)
  Integrator2 : Integrator  InitialCondition=zeros(n,1)
  Integrator3 : Integrator  ExternalReset=level  InitialCondition=zeros(n,1)
  Memory : Memory  InitialCondition=zeros(n,1)
  Memory1 : Memory  InitialCondition=zeros(3,1)
  Sum : Sum  Inputs=|++
  g-Estimator : MATLAB Function  TreatAsAtomicUnit=on
  g-Estimator1 : MATLAB Function  TreatAsAtomicUnit=on
  main : MATLAB Function  TreatAsAtomicUnit=on
  output definition : MATLAB Function  TreatAsAtomicUnit=on
  variable change : MATLAB Function  TreatAsAtomicUnit=on
  N1 : Outport
  wires:
  x_rd/1 -> variable change/2(Xd)
  X/1 -> variable change/1(X)
  CARE/1(DP) -> Integrator1/1
  Sum/1 -> main/1(sigma), g-Estimator/1(sigma), g-Estimator1/1(sigma)
  g-Estimator1/1(Da_hat) -> Integrator/1
  variable change/1(x_mod) -> main/7(x), g-Estimator1/2(x)
  Integrator1/1 -> g-Estimator1/3(P), CARE/1(P), g-Estimator/3(P), main/4(P)
  Integrator/1 -> g-Estimator1/4(a_hat), CARE/2(a_hat), main/5(a_hat)
  g-Estimator/1(Dg_hat) -> Integrator2/1
  Differentiator/1(Dx_d) -> main/3(Dy_d)
  Integrator3/1 -> main/2(zeta), Sum/1
  variable change/2(xd_mod) -> Differentiator/1(x_d)
  variable change/3(e_mod) -> Sum/2, Integrator3/2, Integrator3/1
  Integrator2/1 -> main/6(g_hat), g-Estimator/2(g_hat)
  output definition/1(ur) -> Memory1/1
  Memory1/1 -> N1/1
  main/1(u) -> output definition/1(u), Memory/1
  Memory/1 -> variable change/3(u)

== system Simple_4Quad_payload_08_2017b/Controllers and Observers/Cotnroller and Observer - Agent1 /Observer1 ==
  wo : Inport
  Dwo : Inport  Port=2
  Rel_Pos_local1 : Inport  Port=3
  Rel_Acc_local1 : Inport  Port=4
  Agent_Num : Inport  Port=5
  Integrator : Integrator  InitialCondition=eye(6)
  Integrator1 : Integrator  InitialCondition=[0;0;1;0;0;0]
  Kalman_Filter1 : MATLAB Function  TreatAsAtomicUnit=on
  Observer_Finalization1 : MATLAB Function  TreatAsAtomicUnit=on
  q1_hat : Outport
  Dq1_hat : Outport  Port=2
  tag scope: Dq1_hat=global, q1_hat=global
  wires:
  Kalman_Filter1/1(DP_ob) -> Integrator/1
  Kalman_Filter1/2(Dxhat_ob) -> Integrator1/1
  Integrator/1 -> Kalman_Filter1/1(P_ob)
  Integrator1/1 -> Observer_Finalization1/1(xhati), Kalman_Filter1/2(xhat_ob)
  wo/1 -> Kalman_Filter1/3(wo)
  Dwo/1 -> Kalman_Filter1/4(Dwo)
  Rel_Pos_local1/1 -> Kalman_Filter1/5(Rel_Posi_local)
  Rel_Acc_local1/1 -> Kalman_Filter1/6(Rel_Acci_local)
  Agent_Num/1 -> Kalman_Filter1/7(Agent_Num)
  Observer_Finalization1/1(qhati) -> [q1_hat], q1_hat/1
  Observer_Finalization1/2(Dqhati) -> [Dq1_hat], Dq1_hat/1

== system Simple_4Quad_payload_08_2017b/Controllers and Observers/Cotnroller and Observer - Agent1 /Rotational #1 ==
  x_rd : Inport
  X : Inport  Port=2
  CARE : MATLAB Function  TreatAsAtomicUnit=on
  Differentiator : Subsystem
  Integrator : Integrator  InitialCondition=zeros(n)
  Integrator1 : Integrator  InitialCondition=eye(n)
  Integrator2 : Integrator  InitialCondition=zeros(n,1)
  Integrator3 : Integrator  InitialCondition=zeros(n,1)
  Memory : Memory  InitialCondition=zeros(n,1)
  Memory1 : Memory  InitialCondition=zeros(3,1)
  Sum : Sum  Inputs=|++
  g-Estimator : MATLAB Function  TreatAsAtomicUnit=on
  g-Estimator1 : MATLAB Function  TreatAsAtomicUnit=on
  main : MATLAB Function  TreatAsAtomicUnit=on
  output definition : MATLAB Function  TreatAsAtomicUnit=on
  variable change : MATLAB Function  TreatAsAtomicUnit=on
  ur1 : Outport
  tag scope: A_hat1_R=global, P1_R=global, e1_R=global, g_hat1_R=global
  wires:
  x_rd/1 -> variable change/2(Xd)
  X/1 -> variable change/1(X)
  CARE/1(DP) -> Integrator1/1
  Sum/1 -> main/1(sigma), g-Estimator/1(sigma), g-Estimator1/1(sigma)
  g-Estimator1/1(Da_hat) -> Integrator/1
  variable change/1(x_mod) -> main/7(x), g-Estimator1/2(x)
  Integrator1/1 -> g-Estimator1/3(P), CARE/1(P), [P1_R], g-Estimator/3(P), main/4(P)
  Integrator/1 -> [A_hat1_R], g-Estimator1/4(a_hat), CARE/2(a_hat), main/5(a_hat)
  g-Estimator/1(Dg_hat) -> Integrator2/1
  Differentiator/1(Dx_d) -> main/3(Dy_d)
  Integrator3/1 -> main/2(zeta), Sum/1
  variable change/2(xd_mod) -> Differentiator/1(x_d)
  variable change/3(e_mod) -> [e1_R], Sum/2, Integrator3/1
  Integrator2/1 -> main/6(g_hat), [g_hat1_R], g-Estimator/2(g_hat)
  output definition/1(ur) -> Memory1/1
  Memory1/1 -> ur1/1
  main/1(u) -> output definition/1(u), Memory/1
  Memory/1 -> variable change/3(u)

== system Simple_4Quad_payload_08_2017b/Dynamic model of the entire system/Control inputs from Q1/Rotation_Q1 ==
  Omega Q1 : Inport
  D Phi : MATLAB Function  TreatAsAtomicUnit=on
  Integrator : Integrator  InitialCondition=zeros(3,1)
  Mux : Mux  Inputs=2
  X_Rot_Q1 : Outport
  PHI_Q1 : Outport  Port=2
  wires:
  D Phi/1(D_PHI_Q1) -> Integrator/1
  Omega Q1/1 -> D Phi/1(Omega_Q1), Mux/2
  Integrator/1 -> PHI_Q1/1, D Phi/2(PHI_Q1), Mux/1
  Mux/1 -> X_Rot_Q1/1

== system Simple_4Quad_payload_08_2017b/Dynamic model of the entire system/Control inputs from Q2/Rotation_Q2 ==
  Omega Q2 : Inport
  D Phi : MATLAB Function  TreatAsAtomicUnit=on
  Integrator : Integrator  InitialCondition=zeros(3,1)
  Mux : Mux  Inputs=2
  X_Rot_Q2 : Outport
  PHI_Q2 : Outport  Port=2
  wires:
  D Phi/1(D_PHI_Q2) -> Integrator/1
  Omega Q2/1 -> Mux/2, D Phi/1(Omega_Q2)
  Integrator/1 -> PHI_Q2/1, D Phi/2(PHI_Q2), Mux/1
  Mux/1 -> X_Rot_Q2/1

== system Simple_4Quad_payload_08_2017b/Dynamic model of the entire system/Control inputs from Q3/Rotation_Q3 ==
  Omega Q3 : Inport
  D Phi : MATLAB Function  TreatAsAtomicUnit=on
  Integrator : Integrator  InitialCondition=zeros(3,1)
  Mux : Mux  Inputs=2
  X_Rot_Q3 : Outport
  PHI_Q3 : Outport  Port=2
  wires:
  D Phi/1(D_PHI_Q3) -> Integrator/1
  Omega Q3/1 -> Mux/2, D Phi/1(Omega_Q3)
  Integrator/1 -> PHI_Q3/1, D Phi/2(PHI_Q3), Mux/1
  Mux/1 -> X_Rot_Q3/1

== system Simple_4Quad_payload_08_2017b/Dynamic model of the entire system/Control inputs from Q4/Rotation_Q4 ==
  Omega Q4 : Inport
  D Phi : MATLAB Function  TreatAsAtomicUnit=on
  Integrator : Integrator  InitialCondition=zeros(3,1)
  Mux : Mux  Inputs=2
  X_Rot_Q4 : Outport
  PHI_Q4 : Outport  Port=2
  wires:
  D Phi/1(D_PHI_Q4) -> Integrator/1
  Integrator/1 -> PHI_Q4/1, D Phi/2(PHI_Q4), Mux/1
  Mux/1 -> X_Rot_Q4/1
  Omega Q4/1 -> D Phi/1(Omega_Q4), Mux/2

== system Simple_4Quad_payload_08_2017b/Controllers and Observers/Controlelr and Observer - Agent3/Link #3/Differentiator ==
  x_d : Inport
  Integrator : Integrator  InitialCondition=zeros(n,1)
  Integrator1 : Integrator  InitialCondition=zeros(n,1)
  Sliding differentiator : MATLAB Function  TreatAsAtomicUnit=on
  Sliding differentiator1 : MATLAB Function  TreatAsAtomicUnit=on
  Sum : Sum  Inputs=|-+
  Dx_d : Outport
  wires:
  Sliding differentiator/1(u) -> Integrator1/1, Dx_d/1
  Sliding differentiator1/1(Du1) -> Integrator/1
  Integrator/1 -> Sliding differentiator/1(u1)
  x_d/1 -> Sum/1
  Sum/1 -> Sliding differentiator/2(e), Sliding differentiator1/1(e)
  Integrator1/1 -> Sum/2

== system Simple_4Quad_payload_08_2017b/Controllers and Observers/Controlelr and Observer - Agent3/Rotational #3/Differentiator ==
  x_d : Inport
  Integrator : Integrator  InitialCondition=zeros(n,1)
  Integrator1 : Integrator  InitialCondition=zeros(n,1)
  Scope : Scope
  Scope1 : Scope
  Sliding differentiator : MATLAB Function  TreatAsAtomicUnit=on
  Sliding differentiator1 : MATLAB Function  TreatAsAtomicUnit=on
  Sum : Sum  Inputs=|-+
  Dx_d : Outport
  wires:
  Integrator1/1 -> Sum/2
  Sum/1 -> Sliding differentiator1/1(e), Sliding differentiator/2(e), Scope1/1
  x_d/1 -> Sum/1
  Integrator/1 -> Sliding differentiator/1(u1)
  Sliding differentiator1/1(Du1) -> Integrator/1
  Sliding differentiator/1(u) -> Dx_d/1, Integrator1/1, Scope/1

== system Simple_4Quad_payload_08_2017b/Controllers and Observers/Controller - Payload/Payload/Differentiator ==
  x_d : Inport
  Integrator : Integrator  InitialCondition=zeros(n,1)
  Integrator1 : Integrator  InitialCondition=zeros(n,1)
  Sliding differentiator : MATLAB Function  TreatAsAtomicUnit=on
  Sliding differentiator1 : MATLAB Function  TreatAsAtomicUnit=on
  Sum : Sum  Inputs=|-+
  Dx_d : Outport
  wires:
  Sliding differentiator/1(u) -> Integrator1/1, Dx_d/1
  Sliding differentiator1/1(Du1) -> Integrator/1
  Integrator/1 -> Sliding differentiator/1(u1)
  x_d/1 -> Sum/1
  Sum/1 -> Sliding differentiator/2(e), Sliding differentiator1/1(e)
  Integrator1/1 -> Sum/2

== system Simple_4Quad_payload_08_2017b/Controllers and Observers/Controller - Payload/Payload1/Differentiator ==
  x_d : Inport
  Integrator : Integrator  InitialCondition=zeros(n,1)
  Integrator1 : Integrator  InitialCondition=zeros(n,1)
  Sliding differentiator : MATLAB Function  TreatAsAtomicUnit=on
  Sliding differentiator1 : MATLAB Function  TreatAsAtomicUnit=on
  Sum : Sum  Inputs=|-+
  Dx_d : Outport
  wires:
  Sliding differentiator/1(u) -> Integrator1/1, Dx_d/1
  Sliding differentiator1/1(Du1) -> Integrator/1
  Integrator/1 -> Sliding differentiator/1(u1)
  x_d/1 -> Sum/1
  Sum/1 -> Sliding differentiator/2(e), Sliding differentiator1/1(e)
  Integrator1/1 -> Sum/2

== system Simple_4Quad_payload_08_2017b/Controllers and Observers/Controller and Observer - Agent2/Link #2/Differentiator ==
  x_d : Inport
  Integrator : Integrator  InitialCondition=zeros(n,1)
  Integrator1 : Integrator  InitialCondition=zeros(n,1)
  Sliding differentiator : MATLAB Function  TreatAsAtomicUnit=on
  Sliding differentiator1 : MATLAB Function  TreatAsAtomicUnit=on
  Sum : Sum  Inputs=|-+
  Dx_d : Outport
  wires:
  Sliding differentiator/1(u) -> Integrator1/1, Dx_d/1
  Sliding differentiator1/1(Du1) -> Integrator/1
  Integrator/1 -> Sliding differentiator/1(u1)
  x_d/1 -> Sum/1
  Sum/1 -> Sliding differentiator/2(e), Sliding differentiator1/1(e)
  Integrator1/1 -> Sum/2

== system Simple_4Quad_payload_08_2017b/Controllers and Observers/Controller and Observer - Agent2/Rotational #2/Differentiator ==
  x_d : Inport
  Integrator : Integrator  InitialCondition=zeros(n,1)
  Integrator1 : Integrator  InitialCondition=zeros(n,1)
  Scope : Scope
  Scope1 : Scope
  Sliding differentiator : MATLAB Function  TreatAsAtomicUnit=on
  Sliding differentiator1 : MATLAB Function  TreatAsAtomicUnit=on
  Sum : Sum  Inputs=|-+
  Dx_d : Outport
  wires:
  Sliding differentiator/1(u) -> Scope/1, Integrator1/1, Dx_d/1
  Sliding differentiator1/1(Du1) -> Integrator/1
  Integrator/1 -> Sliding differentiator/1(u1)
  x_d/1 -> Sum/1
  Sum/1 -> Scope1/1, Sliding differentiator/2(e), Sliding differentiator1/1(e)
  Integrator1/1 -> Sum/2

== system Simple_4Quad_payload_08_2017b/Controllers and Observers/Controller and Observer - Agent4/Link #4/Differentiator ==
  x_d : Inport
  Integrator : Integrator  InitialCondition=zeros(n,1)
  Integrator1 : Integrator  InitialCondition=zeros(n,1)
  Sliding differentiator : MATLAB Function  TreatAsAtomicUnit=on
  Sliding differentiator1 : MATLAB Function  TreatAsAtomicUnit=on
  Sum : Sum  Inputs=|-+
  Dx_d : Outport
  wires:
  Sliding differentiator/1(u) -> Integrator1/1, Dx_d/1
  Sliding differentiator1/1(Du1) -> Integrator/1
  Integrator/1 -> Sliding differentiator/1(u1)
  x_d/1 -> Sum/1
  Sum/1 -> Sliding differentiator/2(e), Sliding differentiator1/1(e)
  Integrator1/1 -> Sum/2

== system Simple_4Quad_payload_08_2017b/Controllers and Observers/Controller and Observer - Agent4/Rotational #4/Differentiator ==
  x_d : Inport
  Integrator : Integrator  InitialCondition=zeros(n,1)
  Integrator1 : Integrator  InitialCondition=zeros(n,1)
  Scope : Scope
  Scope1 : Scope
  Sliding differentiator : MATLAB Function  TreatAsAtomicUnit=on
  Sliding differentiator1 : MATLAB Function  TreatAsAtomicUnit=on
  Sum : Sum  Inputs=|-+
  Dx_d : Outport
  wires:
  Sliding differentiator/1(u) -> Scope/1, Integrator1/1, Dx_d/1
  Sliding differentiator1/1(Du1) -> Integrator/1
  Integrator/1 -> Sliding differentiator/1(u1)
  x_d/1 -> Sum/1
  Sum/1 -> Scope1/1, Sliding differentiator/2(e), Sliding differentiator1/1(e)
  Integrator1/1 -> Sum/2

== system Simple_4Quad_payload_08_2017b/Controllers and Observers/Cotnroller and Observer - Agent1 /Link #1/Differentiator ==
  x_d : Inport
  Integrator : Integrator  InitialCondition=zeros(n,1)
  Integrator1 : Integrator  InitialCondition=zeros(n,1)
  Sliding differentiator : MATLAB Function  TreatAsAtomicUnit=on
  Sliding differentiator1 : MATLAB Function  TreatAsAtomicUnit=on
  Sum : Sum  Inputs=|-+
  Dx_d : Outport
  wires:
  Sliding differentiator/1(u) -> Integrator1/1, Dx_d/1
  Sliding differentiator1/1(Du1) -> Integrator/1
  Integrator/1 -> Sliding differentiator/1(u1)
  x_d/1 -> Sum/1
  Sum/1 -> Sliding differentiator/2(e), Sliding differentiator1/1(e)
  Integrator1/1 -> Sum/2

== system Simple_4Quad_payload_08_2017b/Controllers and Observers/Cotnroller and Observer - Agent1 /Rotational #1/Differentiator ==
  x_d : Inport
  Integrator : Integrator  InitialCondition=zeros(n,1)
  Integrator1 : Integrator  InitialCondition=zeros(n,1)
  Sliding differentiator : MATLAB Function  TreatAsAtomicUnit=on
  Sliding differentiator1 : MATLAB Function  TreatAsAtomicUnit=on
  Sum : Sum  Inputs=|-+
  Dx_d : Outport
  wires:
  Sliding differentiator/1(u) -> Integrator1/1, Dx_d/1
  Sliding differentiator1/1(Du1) -> Integrator/1
  Integrator/1 -> Sliding differentiator/1(u1)
  x_d/1 -> Sum/1
  Sum/1 -> Sliding differentiator/2(e), Sliding differentiator1/1(e)
  Integrator1/1 -> Sum/2
